simulink model "OBSTACLEAVOIDANCE"  (R2023b)
settings: Solver=VariableStepAuto  StartTime=0.0  StopTime=10.0  RelTol=1e-3
settings Model: Creator=lucaerviati  LastModifiedBy=carol
settings OptimizationCC: ReuseModelBlockBuffer=off

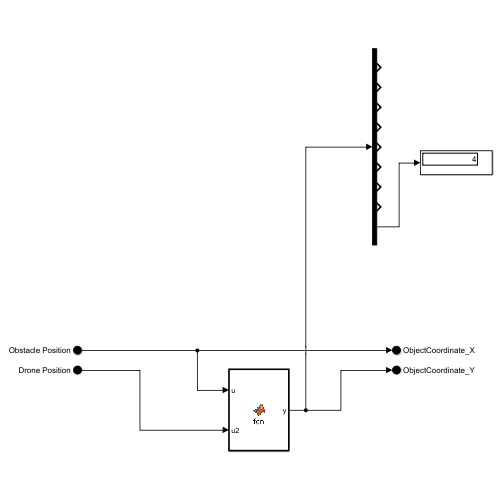
[thumbnail: Simulink's stored preview of the top-level diagram]
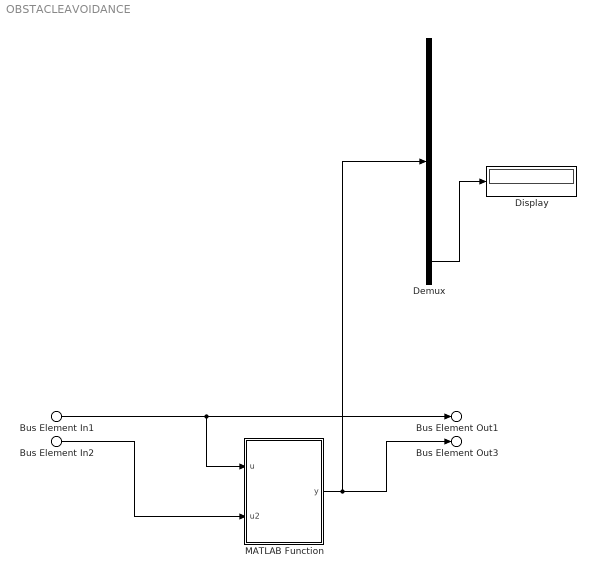
== system OBSTACLEAVOIDANCE ==
  Bus Element In1 : Inport  PortName=Obstacle Position
  Bus Element In2 : Inport  Port=2  PortName=Drone Position
  Demux : Demux  Outputs=9
  Display : Display
  MATLAB Function : MATLAB Function  TreatAsAtomicUnit=on
  Bus Element Out1 : Outport  PortName=ObjectCoordinate_X
  Bus Element Out3 : Outport  Port=2  PortName=ObjectCoordinate_Y
  wires:
  Bus Element In1/1 -> MATLAB Function/1(u), Bus Element Out1/1
  MATLAB Function/1(y) -> Demux/1, Bus Element Out3/1
  Bus Element In2/1 -> MATLAB Function/2(u2)
  Demux/9 -> Display/1

== matlab function OBSTACLEAVOIDANCE/MATLAB Function ==
  data: u input; y output; u2 input
function y = fcn(u,u2)

u = rand(1);
if u>0.5
    y = [1,2,30,4,1,1,12,3,4];
else
    y = [0,2,30,4,1,1,12,3,4];
end
